simulink model "Openloop_voltage_control"  (R2020b)
settings: Solver=FixedStepDiscrete  StartTime=0.0  StopTime=Inf  RelTol=1e-3  EnableMultiTasking=on
values from neighbouring files (symbols this model uses):
  D_IGBT_CCM = (V_IGBT_out+V_diode_forward_drop-V_in)/(V_IGBT_out+V_diode_forward_drop)    (= 0.850746268657)    [Openloop_voltage_control_parameters.m]
  D_MOSFET_CCM = (V_MOSFET_out+V_diode_forward_drop-V_in)/(V_MOSFET_out+V_diode_forward_drop)    (= 0.70297029703)    [Openloop_voltage_control_parameters.m]
  Ki_IGBT = 0    [Openloop_voltage_control_parameters.m]
  Ki_MOSFET = 0    [Openloop_voltage_control_parameters.m]
  Kp_IGBT = 0    [Openloop_voltage_control_parameters.m]
  Kp_MOSFET = 0    [Openloop_voltage_control_parameters.m]
  Timer_period_IGBT = round(60e6/f_sw_IGBT)    [Openloop_voltage_control_parameters.m]
  Timer_period_MOSFET = round(60e6/f_sw_MOSFET)    [Openloop_voltage_control_parameters.m]
undefined symbols (not defined in the file or in its folder): GPTRIP1SEL, GPTRIP2SEL, TZ1, TZ2
undefined symbols (not defined in the file): C2000, Clear, Disable, ePWM2, ePWMxA, Immediate, Positive, Set, Up
libraries: c2802xlib x9, pid_lib x2, dspsigops x2, c280xlib x1
(part 2 of 2)

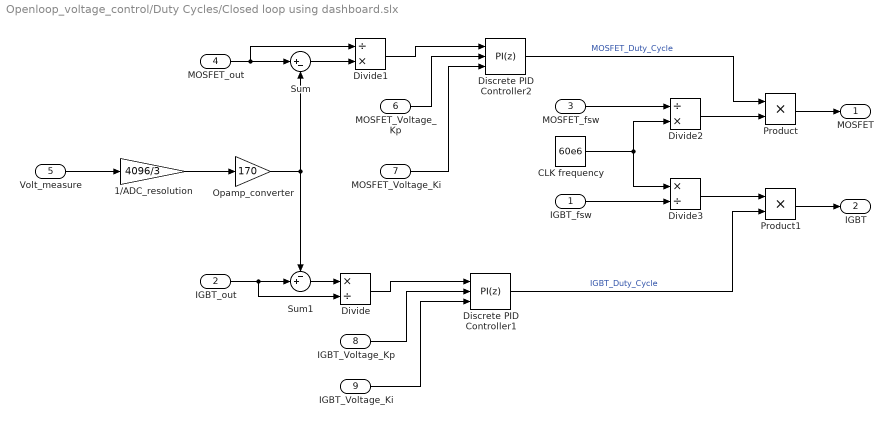
== system Openloop_voltage_control/Duty Cycles/Closed loop using dashboard.slx ==
  IGBT_fsw : Inport
  IGBT_out : Inport  Port=2
  MOSFET_fsw : Inport  Port=3
  MOSFET_out : Inport  Port=4
  Volt_measure : Inport  Port=5
  MOSFET_Voltage_Kp : Inport  Port=6
  MOSFET_Voltage_Ki : Inport  Port=7
  IGBT_Voltage_Kp : Inport  Port=8
  IGBT_Voltage_Ki : Inport  Port=9
  1/ADC_resolution : Gain  Gain=4096/3
  CLK frequency : Constant  Value=60e6
  Discrete PID Controller1 : pid_lib/PID Controller  Controller=PI  Form=Parallel  TimeDomain=Discrete-time  UseExternalTs=off  SampleTime=-1  IntegratorMethod=Forward Euler  FilterMethod=Forward Euler  ControllerParametersSource=external  P=Kp_IGBT  I=Ki_IGBT  D=0  UseFilter=on  N=100  TunerSelectOption=Transfer Function Based (PID Tuner App)  InitialConditionSource=internal  InitialConditionForIntegrator=0  InitialConditionForFilter=0  DifferentiatorICPrevScaledInput=0  ExternalReset=none  TrackingMode=off  Kt=1  LimitOutput=off  SatLimitsSource=internal  UpperSaturationLimit=600  LowerSaturationLimit=-5  LinearizeAsGain=off  AntiWindupMode=clamping  Kb=1  POutMin=[]  POutMax=[]  IOutMin=[]  IOutMax=[]  DOutMin=[]  DOutMax=[]  NOutMin=[]  NOutMax=[]  SumOutMin=[]  SumOutMax=[]  SaturationOutMin=[]  SaturationOutMax=[]  PParamMin=[]  PParamMax=[]  IParamMin=[]  IParamMax=[]  DParamMin=[]  DParamMax=[]  NParamMin=[]  NParamMax=[]  KbParamMin=[]  KbParamMax=[]  KtParamMin=[]  KtParamMax=[]  KbOutMin=[]  KbOutMax=[]  KtOutMin=[]  KtOutMax=[]  IntegratorOutMin=[]  IntegratorOutMax=[]  FilterOutMin=[]  FilterOutMax=[]  SumI1OutMin=[]  SumI1OutMax=[]  SumI2OutMin=[]  SumI2OutMax=[]  SumI3OutMin=[]  SumI3OutMax=[]  SumI4OutMin=[]  SumI4OutMax=[]  SumDOutMin=[]  SumDOutMax=[]  DifferentiatorOutMin=[]  DifferentiatorOutMax=[]  FilterDiffOutCoefMin=[]  FilterDiffOutCoefMax=[]  ReciprocalOutMin=[]  ReciprocalOutMax=[]  SumDenOutMin=[]  SumDenOutMax=[]  SumNumOutMin=[]  SumNumOutMax=[]  DivideOutMin=[]  DivideOutMax=[]  UdiffTsProdOutMin=[]  UdiffTsProdOutMax=[]  NTsProdOutMin=[]  NTsProdOutMax=[]  UintegralTsProdOutMin=[]  UintegralTsProdOutMax=[]  UngainTsProdOutMin=[]  UngainTsProdOutMax=[]  IntegratorContinuousStateAttributes=''  IntegratorStateMustResolveToSignalObject=off  IntegratorRTWStateStorageClass=Auto  FilterContinuousStateAttributes=''  FilterStateMustResolveToSignalObject=off  FilterRTWStateStorageClass=Auto  ParallelPVariant=ExternalParameters  IdealPVariant=Disabled  IVariant=ExternalParameters  DVariant=Disabled  IntegratorVariant=Discrete  SatVariant=Disabled  AWVariant=Passthrough  PCopyVariant=Disabled  TRVariant=Disabled  FdbkBlocksVariant=Forward  IdealPFdbkVariant=Disabled  SatFdbkVariant=Disabled  DerivativeFilterVariant=Disabled  NVariant=Disabled  NCopyVariant=Disabled_SignalSpec  FilterICVariant=Disabled  IntegratorICVariant=InternalICs  ExternalResetVariant=Disabled  TRSumVariant=Passthrough  SumFdbkVariant=Disabled  SumVariant=Sum_PI  TsampFilterVariant=InternalTs  TsampNgainVariant=Passthrough  TsampIntegralVariant=Passthrough  ExternalSaturationOutDataTypeStr=Inherit: Same as second input
  Discrete PID Controller2 : pid_lib/PID Controller  Controller=PI  Form=Parallel  TimeDomain=Discrete-time  UseExternalTs=off  SampleTime=-1  IntegratorMethod=Forward Euler  FilterMethod=Forward Euler  ControllerParametersSource=external  P=Kp_MOSFET  I=Ki_MOSFET  D=0  UseFilter=on  N=100  TunerSelectOption=Transfer Function Based (PID Tuner App)  InitialConditionSource=internal  InitialConditionForIntegrator=0  InitialConditionForFilter=0  DifferentiatorICPrevScaledInput=0  ExternalReset=none  TrackingMode=off  Kt=1  LimitOutput=off  SatLimitsSource=internal  UpperSaturationLimit=600  LowerSaturationLimit=-5  LinearizeAsGain=off  AntiWindupMode=none  Kb=1  POutMin=[]  POutMax=[]  IOutMin=[]  IOutMax=[]  DOutMin=[]  DOutMax=[]  NOutMin=[]  NOutMax=[]  SumOutMin=[]  SumOutMax=[]  SaturationOutMin=[]  SaturationOutMax=[]  PParamMin=[]  PParamMax=[]  IParamMin=[]  IParamMax=[]  DParamMin=[]  DParamMax=[]  NParamMin=[]  NParamMax=[]  KbParamMin=[]  KbParamMax=[]  KtParamMin=[]  KtParamMax=[]  KbOutMin=[]  KbOutMax=[]  KtOutMin=[]  KtOutMax=[]  IntegratorOutMin=[]  IntegratorOutMax=[]  FilterOutMin=[]  FilterOutMax=[]  SumI1OutMin=[]  SumI1OutMax=[]  SumI2OutMin=[]  SumI2OutMax=[]  SumI3OutMin=[]  SumI3OutMax=[]  SumI4OutMin=[]  SumI4OutMax=[]  SumDOutMin=[]  SumDOutMax=[]  DifferentiatorOutMin=[]  DifferentiatorOutMax=[]  FilterDiffOutCoefMin=[]  FilterDiffOutCoefMax=[]  ReciprocalOutMin=[]  ReciprocalOutMax=[]  SumDenOutMin=[]  SumDenOutMax=[]  SumNumOutMin=[]  SumNumOutMax=[]  DivideOutMin=[]  DivideOutMax=[]  UdiffTsProdOutMin=[]  UdiffTsProdOutMax=[]  NTsProdOutMin=[]  NTsProdOutMax=[]  UintegralTsProdOutMin=[]  UintegralTsProdOutMax=[]  UngainTsProdOutMin=[]  UngainTsProdOutMax=[]  IntegratorContinuousStateAttributes=''  IntegratorStateMustResolveToSignalObject=off  IntegratorRTWStateStorageClass=Auto  FilterContinuousStateAttributes=''  FilterStateMustResolveToSignalObject=off  FilterRTWStateStorageClass=Auto  ParallelPVariant=ExternalParameters  IdealPVariant=Disabled  IVariant=ExternalParameters  DVariant=Disabled  IntegratorVariant=Discrete  SatVariant=Disabled  AWVariant=Passthrough  PCopyVariant=Disabled  TRVariant=Disabled  FdbkBlocksVariant=Forward  IdealPFdbkVariant=Disabled  SatFdbkVariant=Disabled  DerivativeFilterVariant=Disabled  NVariant=Disabled  NCopyVariant=Disabled_SignalSpec  FilterICVariant=Disabled  IntegratorICVariant=InternalICs  ExternalResetVariant=Disabled  TRSumVariant=Passthrough  SumFdbkVariant=Disabled  SumVariant=Sum_PI  TsampFilterVariant=InternalTs  TsampNgainVariant=Passthrough  TsampIntegralVariant=Passthrough  ExternalSaturationOutDataTypeStr=Inherit: Same as second input
  Divide : Product  Inputs=*/
  Divide1 : Product  Inputs=/*
  Divide2 : Product  Inputs=/*
  Divide3 : Product  Inputs=*/
  Opamp_converter : Gain  Gain=170
  Product : Product
  Product1 : Product
  Sum : Sum  Inputs=|+-
  Sum1 : Sum  Inputs=-+|
  MOSFET : Outport
  IGBT : Outport  Port=2
  wires:
  MOSFET_out/1 -> Sum/1, Divide1/1
  Sum1/1 -> Divide/1
  Divide1/1 -> Discrete PID Controller2/1
  Sum/1 -> Divide1/2
  Divide/1 -> Discrete PID Controller1/1
  IGBT_out/1 -> Sum1/2, Divide/2
  Discrete PID Controller1/1 -> Product1/2  "IGBT_Duty_Cycle"
  Discrete PID Controller2/1 -> Product/1  "MOSFET_Duty_Cycle"
  MOSFET_fsw/1 -> Divide2/1
  Divide3/1 -> Product1/1
  Product/1 -> MOSFET/1
  Product1/1 -> IGBT/1
  Divide2/1 -> Product/2
  IGBT_fsw/1 -> Divide3/2
  CLK frequency/1 -> Divide2/2, Divide3/1
  MOSFET_Voltage_Kp/1 -> Discrete PID Controller2/2
  MOSFET_Voltage_Ki/1 -> Discrete PID Controller2/3
  IGBT_Voltage_Kp/1 -> Discrete PID Controller1/2
  IGBT_Voltage_Ki/1 -> Discrete PID Controller1/3
  Opamp_converter/1 -> Sum/2, Sum1/1
  1/ADC_resolution/1 -> Opamp_converter/1
  Volt_measure/1 -> 1/ADC_resolution/1

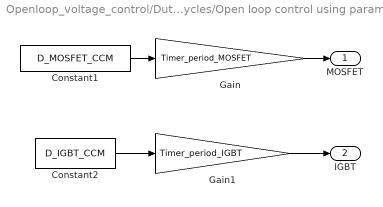
== system Openloop_voltage_control/Duty Cycles/Open loop control using parameter.m ==
  Constant1 : Constant  Value=D_MOSFET_CCM
  Constant2 : Constant  Value=D_IGBT_CCM
  Gain : Gain  Gain=Timer_period_MOSFET
  Gain1 : Gain  Gain=Timer_period_IGBT
  MOSFET : Outport
  IGBT : Outport  Port=2
  wires:
  Constant1/1 -> Gain/1
  Gain/1 -> MOSFET/1
  Constant2/1 -> Gain1/1
  Gain1/1 -> IGBT/1

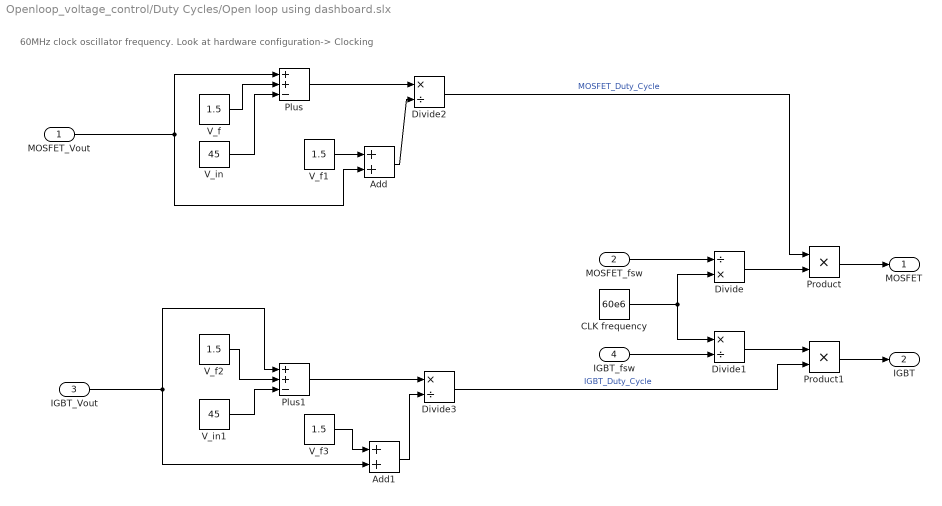
== system Openloop_voltage_control/Duty Cycles/Open loop using dashboard.slx ==
  note: 60MHz clock oscillator frequency. Look at hardware configuration-> Clocking
  MOSFET_Vout : Inport
  MOSFET_fsw : Inport  Port=2
  IGBT_Vout : Inport  Port=3
  IGBT_fsw : Inport  Port=4
  Add : Sum
  Add1 : Sum
  CLK frequency : Constant  Value=60e6
  Divide : Product  Inputs=/*
  Divide1 : Product  Inputs=*/
  Divide2 : Product  Inputs=*/
  Divide3 : Product  Inputs=*/
  Plus : Sum  Inputs=++-
  Plus1 : Sum  Inputs=++-
  Product : Product
  Product1 : Product
  V_f{,1..3} (4 alike) : Constant  Value=1.5
  V_in : Constant  Value=45
  V_in1 : Constant  Value=45
  MOSFET : Outport
  IGBT : Outport  Port=2
  wires:
  Product/1 -> MOSFET/1
  CLK frequency/1 -> Divide/2, Divide1/1
  Add/1 -> Divide2/2
  V_in/1 -> Plus/3
  V_f/1 -> Plus/2
  Plus/1 -> Divide2/1
  Divide/1 -> Product/2
  Divide2/1 -> Product/1  "MOSFET_Duty_Cycle"
  V_f2/1 -> Plus1/2
  Plus1/1 -> Divide3/1
  Add1/1 -> Divide3/2
  Divide3/1 -> Product1/2  "IGBT_Duty_Cycle"
  V_in1/1 -> Plus1/3
  Product1/1 -> IGBT/1
  Divide1/1 -> Product1/1
  V_f1/1 -> Add/1
  V_f3/1 -> Add1/1
  MOSFET_fsw/1 -> Divide/1
  MOSFET_Vout/1 -> Add/2, Plus/1
  IGBT_Vout/1 -> Add1/2, Plus1/1
  IGBT_fsw/1 -> Divide1/2

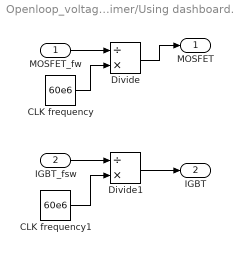
== system Openloop_voltage_control/Timer/Using dashboard.slx ==
  MOSFET_fw : Inport
  IGBT_fsw : Inport  Port=2
  CLK frequency : Constant  Value=60e6
  CLK frequency1 : Constant  Value=60e6
  Divide : Product  Inputs=/*
  Divide1 : Product  Inputs=/*
  MOSFET : Outport
  IGBT : Outport  Port=2
  wires:
  Divide/1 -> MOSFET/1
  Divide1/1 -> IGBT/1
  MOSFET_fw/1 -> Divide/1
  CLK frequency/1 -> Divide/2
  CLK frequency1/1 -> Divide1/2
  IGBT_fsw/1 -> Divide1/1

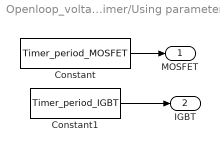
== system Openloop_voltage_control/Timer/Using parameter.m ==
  Constant : Constant  Value=Timer_period_MOSFET
  Constant1 : Constant  Value=Timer_period_IGBT
  MOSFET : Outport
  IGBT : Outport  Port=2
  wires:
  Constant/1 -> MOSFET/1
  Constant1/1 -> IGBT/1

== matlab function Openloop_voltage_control/Logic circuit/MATLAB Function ==
  data: u input; y1 output; y2 output
function [y1,y2]= fcn(u)

if u==0;
    y1=1000;
    y2=1000;
elseif u == 1;
    y1=1000;
    y2=0;
elseif u==2; 
    y1=0;
    y2=1000;
else   
    y1=1000;
    y2=1000;
end
